simulink model "satq_prev_SATQ"  (R2017a)
settings: Solver=VariableStepAuto  StartTime=0.0  StopTime=50.0  RelTol=1e-3
values from neighbouring files (symbols this model uses):
  b = 0.250025    [satq_values.m]
  beta = 0.55    [satq_values.m]
  d = 0.25    [satq_values.m]
  delta = 0.3    [satq_values.m]
  epsilon = 0.8    [satq_values.m]
  N_0 = 1000    [satq_values.m]
settings Model: Creator=rosha  LastModifiedBy=rosha

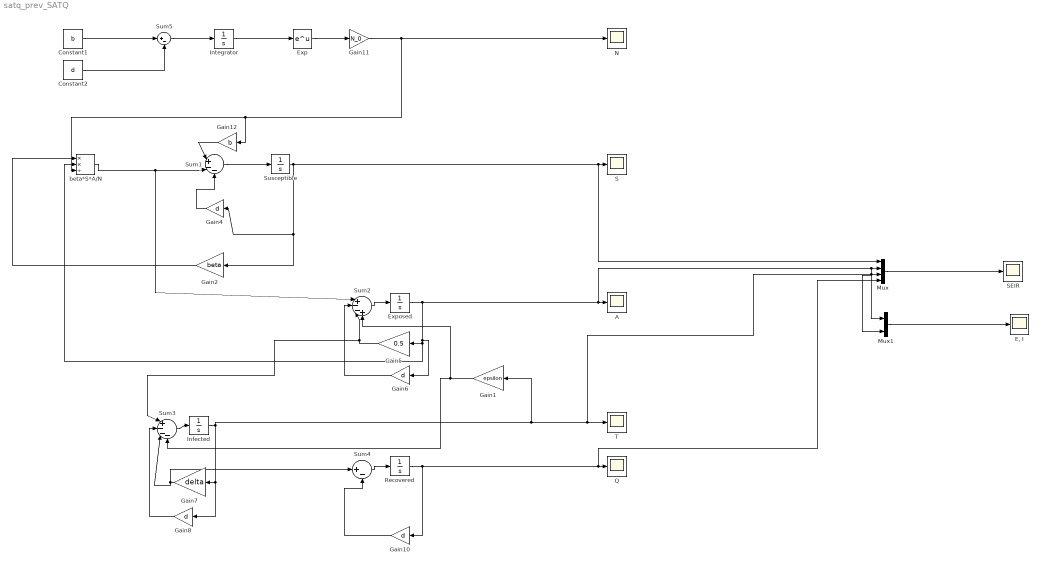
== system satq_prev_SATQ ==
  A : Scope
  Constant1 : Constant  Value=b
  Constant2 : Constant  Value=d
  "E, I" : Scope
  Exp : Math  SaturateOnIntegerOverflow=on
  Exposed : Integrator  InitialCondition=250
  Gain1 : Gain  Gain=epsilon
  Gain{4,6,8,10} (4 alike) : Gain  Gain=d
  Gain11 : Gain  Gain=N_0
  Gain12 : Gain  Gain=b
  Gain2 : Gain  Gain=beta
  Gain5 : Gain  Gain=0.5
  Gain7 : Gain  Gain=delta
  Infected : Integrator  InitialCondition=80
  Integrator : Integrator
  Mux : Mux
  Mux1 : Mux  Inputs=2
  N : Scope
  Q : Scope
  Recovered : Integrator  InitialCondition=20
  S : Scope
  SEIR : Scope
  Sum1 : Sum  Inputs=|+--
  Sum2 : Sum  Inputs=|+--+
  Sum3 : Sum  Inputs=|+---
  Sum4 : Sum  Inputs=|+-
  Sum5 : Sum  Inputs=|+-
  Susceptible : Integrator  InitialCondition=650
  T : Scope
  beta*S*A/N : Product  Inputs=**/
  wires:
  Gain12/1 -> Sum1/1
  Gain7/1 -> Sum3/3, Sum4/1
  Sum4/1 -> Recovered/1
  Gain8/1 -> Sum3/2
  Constant1/1 -> Sum5/1
  Integrator/1 -> Exp/1
  Gain11/1 -> Gain12/1, beta*S*A/N/3, N/1
  Infected/1 -> Gain8/1, Gain7/1, Gain1/1, Mux1/2, Mux/3, T/1
  Sum3/1 -> Infected/1
  Recovered/1 -> Gain10/1, Mux/4, Q/1
  Mux1/1 -> "E, I"/1
  Exposed/1 -> beta*S*A/N/2, Gain5/1, Gain6/1, Mux1/1, Mux/2, A/1
  Gain5/1 -> Sum3/1, Sum2/3
  Sum5/1 -> Integrator/1
  Gain10/1 -> Sum4/2
  Exp/1 -> Gain11/1
  Sum1/1 -> Susceptible/1
  Sum2/1 -> Exposed/1
  Mux/1 -> SEIR/1
  beta*S*A/N/1 -> Sum2/1, Sum1/2
  Constant2/1 -> Sum5/2
  Gain4/1 -> Sum1/3
  Gain2/1 -> beta*S*A/N/1
  Susceptible/1 -> Gain4/1, Gain2/1, Mux/1, S/1
  Gain6/1 -> Sum2/2
  Gain1/1 -> Sum3/4, Sum2/4
